simulink model "Hexapod_Model"  (R2023b)
settings: Solver=FixedStepAuto  StartTime=0.0  StopTime=inf  FixedStep=1  RelTol=1e-3
values from neighbouring files (symbols this model uses):
  button_status = false    [Hexapod_Interface_v1_0.m]
settings Model: Creator=andre  LastModifiedBy=andre
settings OptimizationCC: BlockReduction=off
settings GRTTargetCC: ExtMode=on

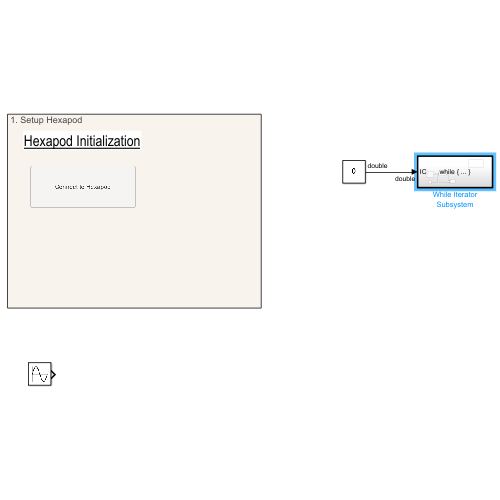
[thumbnail: Simulink's stored preview of the top-level diagram]
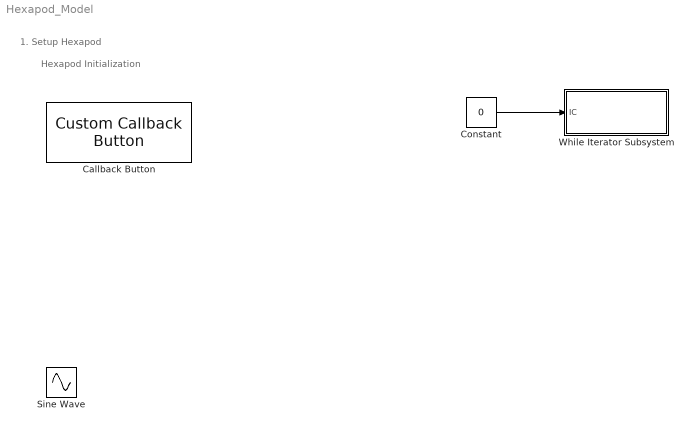
== system Hexapod_Model ==
  note: 1. Setup Hexapod
  note: Hexapod Initialization
  Callback Button : CustomCallbackButton  Configuration="{\"components\":[{\"name\":\"BackgroundImageComponent\",\"settings\":{\"image\":{\"size\":[0,0],\"src\":\"default\",\"srcOrientation\":\"Right\"},\"position\":[0,0,1,1]}},{\"name\":\"ButtonStateComponent\",\"settings\":{\"buttonType\":\"latch\",\"clickFcn\":\"% Connecting to Hexapod thru MATLAB Driver\\n\\ndisp('Connecting to Hexapod')\\n\\nisWindows   = any (strcmp (mexext, {'mexw32', 'mexw64'}));\\n\\nif (isWindows)\\n    matlabDriverPath = getenv ('PI_MATLAB_DRIVER');\\n    if (~exist(matlabDriverPath,'dir'))\\n        error('The PI MATLAB Driver GCS2 was not found on your system. Probably it is not installed. Please run PISoftwareSuite.exe to install the driver.');\\n    else\\n        addpath(matlabDriverPath);\\n    end\\nelse\\n    if (~exist('\\/usr\\/local\\/PI\\/pi_matlab_driver_gcs2','dir'))\\n        error('The PI MATLAB Driver GCS2 was not found on your system. If you need the MATLAB driver for Linux please contact the service.');\\n    else\\n        addpath ('\\/usr\\/local\\/PI\\/pi_matlab_driver_gcs2');\\n    end\\nend\\n\\nif(~exist('Controller','var'))\\n    Controller = PI_GCS_Controller();\\n    Check = true;\\nend\\nif(~isa(Controller,'PI_GCS_Controller'))\\n    Controller = PI_GCS_Controller();\\nend\\n\\nif Check == true\\n    devicesTcpIp = Controller.EnumerateTCPIPDevices();\\n    disp(devicesTcpIp) \\n    stageType = 'C-887.52';\\n    use_TCPIP_Connection = true;\\n    port = 50000;\\n    ip = '169.254.7.214';\\n    C887 = Controller.ConnectTCPIP(ip, port);\\n    C887.qIDN()\\n    C887 = C887.InitializeController();\\nend\\n\\ndisp('Controller Connected')\\n\",\"latched\":false,\"offValue\":null,\"onValue\":1,\"position\":[0,0,1,1],\"pressDelay\":\"500\",\"pressFcn\":\"\",\"repeatInterval\":\"0\",\"states\":[{\"horizontalAlignment\":\"center\",\"image\":{\"position\":[0,0,1,1],\"size\":[1,1],\"src\":\"default\",\"srcOrientation\":\"Right\"},\"label\":{\"color\":[0.01176470588,0.01176470588,0.01176470588,1],\"icon\":{\"size\":[0,0],\"src\":\"default\",\"srcOrientation\":\"Right\"},\"iconPlacement\":\"left\",\"opacity\":1,\"show\":true,\"text\":{\"content\":\"Connect to Hexapod\",\"font\":\"Helvetica\",\"fontSize\":15}},\"labelOffset\":[0,0],\"verticalAlignment\":\"middle\"},{\"horizontalAlignment\":\"center\",\"image\":{\"position\":[0,0,1,1],\"size\":[1,1],\"src\":\"default\",\"srcOrientation\":\"Right\"},\"label\":{\"color\":[0.01176470588,0.01176470588,0.01176470588,1],\"icon\":{\"size\":[0,0],\"src\":\"default\",\"srcOrientation\":\"Right\"},\"iconPlacement\":\"left\",\"opacity\":1,\"show\":true,\"text\":{\"content\":\"Connect to Hexapod\",\"font\":\"Helvetica\",\"fontSize\":15}},\"labelOffset\":[0,0],\"verticalAlignment\":\"middle\"},{\"horizontalAlignment\":\"center\",\"image\":{\"position\":[0,0,1,1],\"size\":[1,1],\"src\":\"default\",\"srcOrientation\":\"Right\"},\"label\":{\"color\":[0.01176470588,0.01176470588,0.01176470588,1],\"icon\":{\"size\":[0,0],\"src\":\"default\",\"srcOrientation\":\"Right\"},\"iconPlacement\":\"left\",\"opacity\":1,\"show\":true,\"text\":{\"content\":\"Connect to Hexapod\",\"font\":\"Helvetica\",\"fontSize\":15}},\"labelOffset\":[0,0],\"verticalAlignment\":\"middle\"},{\"horizontalAlignment\":\"center\",\"image\":{\"position\":[0,0,1,1],\"size\":[1,1],\"src\":\"default\",\"srcOrientation\":\"Right\"},\"label\":{\"color\":[0.01176470588,0.01176470588,0.01176470588,1],\"icon\":{\"size\":[0,0],\"src\":\"default\",\"srcOrientation\":\"Right\"},\"iconPlacement\":\"left\",\"opacity\":1,\"show\":true,\"text\":{\"content\":\"Connect to Hexapod\",\"font\":\"Helvetica\",\"fontSize\":15}},\"labelOffset\":[0,0],\"verticalAlignment\":\"middle\"}]}},{\"name\":\"ForegroundImageComponent\",\"settings\":{\"image\":{\"size\":[0,0],\"src\":\"default\",\"srcOrientation\":\"Right\"},\"isForeground\":1,\"position\":[0,0,1,1]}}],\"settings\":{\"BindingType\":\"standalone\",\"backgroundColor\":[244,244,244,1],\"backgroundOffset\":0.2,\"backgroundOpacity\":1,\"fixedAspectRatio\":\"off\",\"foregroundColor\":[0.01176470588,0.01176470588,0.01176470588,1],\"migratedFromLegacy\":true,\"useBackgroundColor\":true,\"variant\":\"callback\",\"version\":\"R2023a\"},\"type\":\"Button\"}"  CustomBackgroundColor="{\"color\":[0.9568627451,0.9568627451,0.9568627451],\"show\":true}"
  Constant : Constant  Value=0
  Sine Wave : Sin  SampleTime=0
  While Iterator Subsystem : Subsystem  TreatAsAtomicUnit=on
  wires:
  Constant/1 -> While Iterator Subsystem/1(IC)

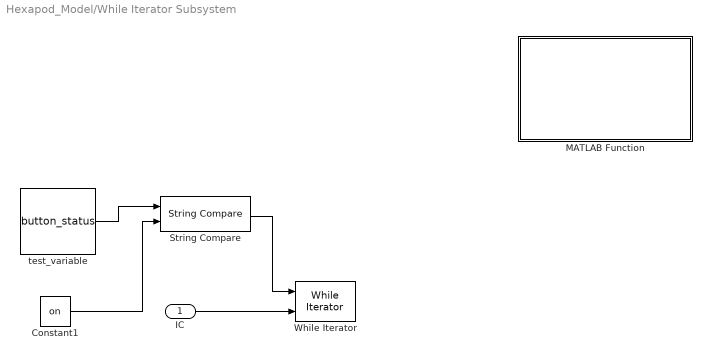
== system Hexapod_Model/While Iterator Subsystem ==
  IC : Inport
  Constant1 : Constant  Value=on
  MATLAB Function : MATLAB Function  TreatAsAtomicUnit=on
  String Compare : StringCompare
  While Iterator : WhileIterator  MaxIters=-1  ResetStates=reset
  test_variable : Constant  Value=button_status
  wires:
  IC/1 -> While Iterator/2
  test_variable/1 -> String Compare/1
  String Compare/1 -> While Iterator/1
  Constant1/1 -> String Compare/2

== matlab function Hexapod_Model/While Iterator Subsystem/MATLAB Function ==
function displayMessage()
% Display a custom message in the MATLAB command window
disp('Hello from Simulink!');


end
